simulink model "w1q5"  (R2019b)
settings: Solver=VariableStepAuto  StartTime=0.0  StopTime=10.0  RelTol=1e-3
settings Model: Creator=Vinayak  LastModifiedBy=Vinayak

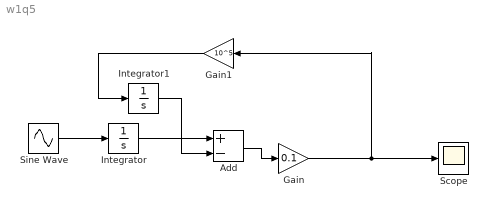
== system w1q5 ==
  Add : Sum  Inputs=+-
  Gain : Gain  Gain=0.1
  Gain1 : Gain  Gain=10^5
  Integrator : Integrator
  Integrator1 : Integrator
  Scope : Scope
  Sine Wave : Sin  SampleTime=0
  wires:
  Sine Wave/1 -> Integrator/1
  Add/1 -> Gain/1
  Gain/1 -> Gain1/1, Scope/1
  Gain1/1 -> Integrator1/1
  Integrator1/1 -> Add/2
  Integrator/1 -> Add/1
